simulink model "ARAI_Academy"  (R2020a)
settings: Solver=FixedStepDiscrete  StartTime=0.0  StopTime=10.0  FixedStep=0.02  RelTol=1e-3
InitFcn:
  | mbd_s32k_consistency_checks(bdroot(gcs));
undefined symbols (not defined in the file): Cells_in_Series, LQFP, Temp_in_Series, ts
libraries: hdlsllib x280, mbd_s32k1xx_ec_toolbox x39, simulink x3
(part 1 of 3)
settings Model: Creator=tg-gr  LastModifiedBy=tg-gr
settings DataIOCC: ExternalInput=off  InitialState=off  SaveOutput=off  SignalLogging=off  SaveTime=off
settings OptimizationCC: DefaultParameterBehavior=Inlined  EnhancedBackFolding=on  PassReuseOutputArgsAs=Individual arguments  ZeroExternalMemoryAtStartup=off  ZeroInternalMemoryAtStartup=off  OptimizeBlockOrder=speed  DifferentSizesBufferReuse=on  OptimizationCustomize=off  EfficientTunableParamExpr=on
settings DebuggingCC: InheritedTsInSrcMsg=none  SingleTaskRateTransMsg=error  ParameterTunabilityLossMsg=error  UnconnectedInputMsg=error  UnconnectedOutputMsg=error  UnconnectedLineMsg=error  UnknownTsInhSupMsg=error
settings HardwareCC: ProdBitPerPointer=32  ProdBitPerSizeT=32  ProdBitPerPtrDiffT=32  ProdLargestAtomicInteger=Long  ProdLargestAtomicFloat=Double  ProdWordSize=32  ProdHWDeviceType=ARM Compatible->ARM Cortex
settings SFSimCC: MATLABDynamicMemAlloc=off
settings RTWCC: Description=Model Based Design Toolbox S32K1xx Code Generation Target  SystemTargetFile=mbd_s32k.tlc  MakeCommand=mbd_s32k_make_rtw COPY_MDLREF_INCLUDES=0  TemplateMakefile=mbd_s32k.tmf
settings CodeAppCC: ForceParamTrailComments=on  IgnoreCustomStorageClasses=off  OperatorAnnotations=on  SimulinkDataObjDesc=on  SFDataObjDesc=on  InsertBlockDesc=on
settings STFCustomTargetCC: TargetLangStandard=C99 (ISO)  MultiwordLength=256  CombineOutputUpdateFcns=on  ERTCustomFileBanners=on  SupportContinuousTime=off  SupportNonInlinedSFcns=off  RemoveResetFunc=on  MATLABClassNameForMDSCustomization=Simulink.SoftwareTarget.ERTCustomization  SystemTargetFile=mbd_s32k.tlc
settings ERTTargetCC: TargetLangStandard=C99 (ISO)  ParMdlRefBuildCompliant=off  CompOptLevelCompliant=off  ConcurrentExecutionCompliant=off  ModelStepFunctionPrototypeControlCompliant=off  CPPClassGenCompliant=off  UseToolchainInfoCompliant=off  InlinedParameterPlacement=NonHierarchical  ERTSrcFileBannerTemplate=mbd_ert_code_template.cgt  ERTHdrFileBannerTemplate=mbd_ert_code_template.cgt  ERTDataSrcFileTemplate=mbd_ert_code_template.cgt  ERTDataHdrFileTemplate=mbd_ert_code_template.cgt  ERTCustomFileTemplate=example_file_process.tlc

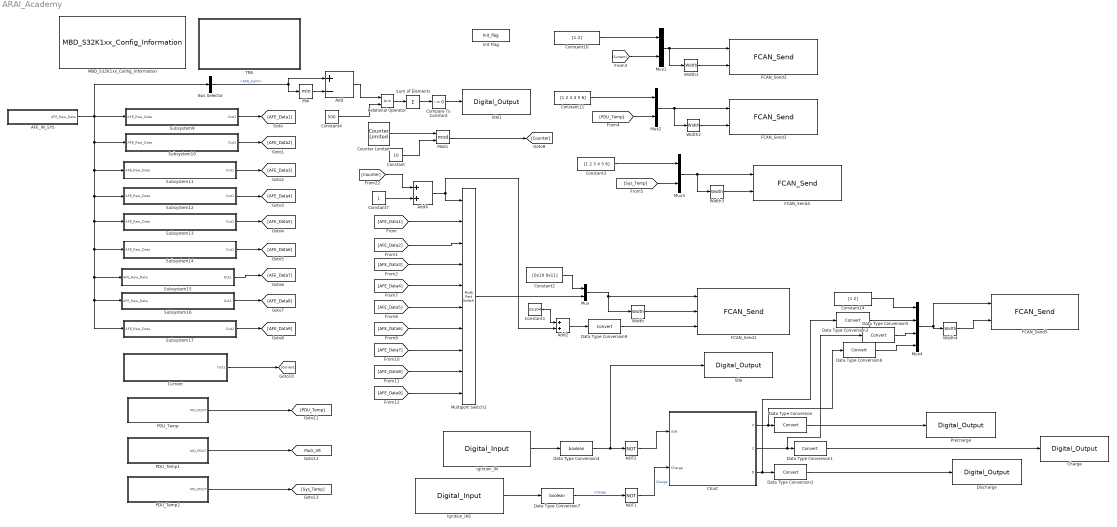
== system ARAI_Academy ==
  AFE_IN_SYS : Subsystem
  Add : Sum  Inputs=+-  OutDataTypeStr=uint16
  Add2 : Sum
  Add4 : Sum
  Bus Selector : BusSelector  OutputSignals=AFE_CellV
  Charge : mbd_s32k1xx_ec_toolbox/GPIO Blocks/Digital_Output  gpio_pin=PTA13: [PTA13 | Port A I/O]  init_val=Low  drive_strength=High
  Chart : Stateflow chart  TreatAsAtomicUnit=on
  Compare To Constant : simulink/Logic and Bit Operations/Compare To Constant  relop=~=  const=0  OutDataTypeStr=boolean
  Constant : Constant  Value=10  OutDataTypeStr=uint8
  Constant1 : Constant  Value=0x104
  Constant10 : Constant  Value=[1 2]  OutDataTypeStr=uint8
  Constant11 : Constant  Value=[1 2 3 4 5 6]  OutDataTypeStr=uint8
  Constant14 : Constant  Value=[1 2]  OutDataTypeStr=uint8
  Constant2 : Constant  Value=[0x10 0x11]
  Constant3 : Constant  Value=[1 2 3 4 5 6]  OutDataTypeStr=uint8
  Constant4 : Constant  Value=500  OutDataTypeStr=uint16
  Constant7 : Constant  OutDataTypeStr=uint8
  Counter Limited : simulink/Sources/Counter Limited  uplimit=8  tsamp=-1
  "Current " : Subsystem
  Data Type Conversion{,1..3,5..6,9} (7 alike) : DataTypeConversion
  Data Type Conversion4 : DataTypeConversion  OutDataTypeStr=boolean
  Data Type Conversion7 : DataTypeConversion  OutDataTypeStr=boolean
  Discharge : mbd_s32k1xx_ec_toolbox/GPIO Blocks/Digital_Output  gpio_pin=PTA12: [PTA12 | Port A I/O]  init_val=Low  drive_strength=High
  FCAN_Send1 : mbd_s32k1xx_ec_toolbox/Communication Blocks/CAN Blocks/FCAN_Send  can_instance=0  can_mode=Non-blocking  can_timeout_ms=0  can_mb_idx=2  can_extended_id=off  can_is_remote=off  can_id=183  show_id_input=on  show_adv_opts=off  can_fd_enable=off  can_enable_brs=off  can_fd_padding=0
  FCAN_Send2 : mbd_s32k1xx_ec_toolbox/Communication Blocks/CAN Blocks/FCAN_Send  can_instance=0  can_mode=Non-blocking  can_timeout_ms=0  can_mb_idx=0  can_extended_id=off  can_is_remote=off  can_id=4  show_id_input=off  show_adv_opts=off  can_fd_enable=off  can_enable_brs=off  can_fd_padding=0
  FCAN_Send3 : mbd_s32k1xx_ec_toolbox/Communication Blocks/CAN Blocks/FCAN_Send  can_instance=0  can_mode=Non-blocking  can_timeout_ms=0  can_mb_idx=1  can_extended_id=off  can_is_remote=off  can_id=1  show_id_input=off  show_adv_opts=off  can_fd_enable=off  can_enable_brs=off  can_fd_padding=0
  FCAN_Send4 : mbd_s32k1xx_ec_toolbox/Communication Blocks/CAN Blocks/FCAN_Send  can_instance=0  can_mode=Non-blocking  can_timeout_ms=0  can_mb_idx=5  can_extended_id=off  can_is_remote=off  can_id=2  show_id_input=off  show_adv_opts=off  can_fd_enable=off  can_enable_brs=off  can_fd_padding=0
  FCAN_Send5 : mbd_s32k1xx_ec_toolbox/Communication Blocks/CAN Blocks/FCAN_Send  can_instance=0  can_mode=Non-blocking  can_timeout_ms=0  can_mb_idx=4  can_extended_id=off  can_is_remote=off  can_id=7  show_id_input=off  show_adv_opts=off  can_fd_enable=off  can_enable_brs=off  can_fd_padding=0
  Idle : mbd_s32k1xx_ec_toolbox/GPIO Blocks/Digital_Output  gpio_pin=PTA11: [PTA11 | Port A I/O]  init_val=Low  drive_strength=High
  Idle1 : mbd_s32k1xx_ec_toolbox/GPIO Blocks/Digital_Output  gpio_pin=PTB9: [PTB9 | Port B I/O]  init_val=Low  drive_strength=High
  Ignition_IN : mbd_s32k1xx_ec_toolbox/GPIO Blocks/Digital_Input  gpio_pin=PTD13: [PTD13 | Port D I/O]  pull_resistor=None  passive_filter=on
  Ignition_IN1 : mbd_s32k1xx_ec_toolbox/GPIO Blocks/Digital_Input  gpio_pin=PTE9: [PTE9 | Port E I/O]  pull_resistor=None  passive_filter=on
  Init Flag : DataStoreMemory  DataStoreName=Init_flag  ReadBeforeWriteMsg=warning  WriteAfterWriteMsg=warning  WriteAfterReadMsg=warning  ShowAdditionalParam=off  OutDataTypeStr=uint8
  MBD_S32K1xx_Config_Information : mbd_s32k1xx_ec_toolbox/MBD_S32K1xx_Config_Information  mbdt_ver=0  disp_str=|  config_params=[]  mcu_target_name=S32K144  mcu_target_package=100-LQFP  mcu_target_sram_size=64KB  mcu_system_clock_freq=80  mcu_xtal_freq=External 8  mcu_steptick_timer=LPIT Channel 0  mcu_steptick_prio=15  ds_import_enable=on  target_compiler=GCC  target_memory=FLASH  gcc_target_compile_opts=-mthumb -mfloat-abi=hard -mfpu=fpv4-sp-d16 -O1 -g -gstrict-dwarf  gcc_target_assemble_opts=-mthumb -mfloat-abi=hard -mfpu=fpv4-sp-d16 -g  gcc_target_link_opts=-mthumb -mfloat-abi=hard -mfpu=fpv4-sp-d16  gcc_target_default_lcf=on  gcc_target_user_lcf=S32K144_64_flash.ld  ghs_target_compile_opts=-cpu=cortexm4f -thumb -fpu=vfpv4_d16 -fsingle -Ogeneral -Wundef -Wimplicit-int -Wshadow -Wtrigraphs --no_commons --gnu_asm -gnu99 -gdwarf-2 -G  ghs_target_assemble_opts=-cpu=cortexm4f -fpu=vfpv4_d16  ghs_target_link_opts=-cpu=cortexm4f -thumb -fpu=vfpv4_d16  ghs_target_default_lcf=on  ghs_target_user_lcf=S32K144_64_flash.ld  iar_target_compile_opts=--cpu=Cortex-M4F --thumb --fpu=VFPv4_sp -Ol -e --debug --dlib_config normal  iar_target_assemble_opts=--cpu Cortex-M4F --thumb --fpu VFPv4_sp  iar_target_link_opts=--no_exceptions --vfe --inline  iar_target_default_lcf=on  iar_target_user_lcf=S32K144_64_flash.icf  pil_download_enable=off  rbl_download_enable=on  rbl_start_delay=5000  rbl_download_interface=OpenSDA  rbl_restart_request=off  rbl_com_port=Custom  rbl_com_port_custom=COM1  pil_download_rate=57600  pil_download_rate_custom=115200  pil_opensda_drive=Custom  pil_opensda_drive_custom=D  jtag_interface=OpenSDA Embedded Debug  pil_uart_instance=1  pil_uart_rx=PTC6: [LPUART1_RX | Receive]  pil_uart_tx=PTC7: [LPUART1_TX | Transmit]  FTM_PWM_PcrCheckEnDis=on  FTM_Input_Edge_Inputs_PcrCheckEnDis=on  FTM_Dual_Edge_Inputs_PcrCheckEnDis=on  FTM_Quadrature_Inputs_PcrCheckEnDis=on  FTM_Hall_Sensor_Inputs_PcrCheckEnDis=on  LPTMR_PcrCheckEnDis=on  PIT_PcrCheckEnDis=on  RTC_PcrCheckEnDis=on  FlexCAN_PcrCheckEnDis=on  LIN_PcrCheckEnDis=on  FlexIO_PcrCheckEnDis=on  LPI2C_PcrCheckEnDis=on  LPSPI_PcrCheckEnDis=on  LPUART_PcrCheckEnDis=on  CMP_PcrCheckEnDis=on  GPIO_OutputPcrCheckEnDis=on  GPIO_InputPcrCheckEnDis=on  SBC_PcrCheckEnDis=on  BMS_PcrCheckEnDis=on  AMMCLIB_PcrCheckEnDis=on  FM_PcrCheckEnDis=on  Profile_PcrCheckEnDis=on  ConfigParams_PcrCheckEnDis=on  ModelRef_PcrCheckEnDis=on  PDB0_PcrCheckEnDis=on  CSEc_PcrCheckEnDis=on  eDMA_PcrCheckEnDis=on  FLASH_PcrCheckEnDis=on  ADC_PcrCheckEnDis=on  WDOG_PcrCheckEnDis=on
      | Target : S32K144-64KB_SRAM
      | Package : 100-pin
      | System clock : 80 MHz
      | XTAL clock : External 8 MHz
      | Compiler : IAR
      | Target Type : FLASH
      | Download Code after build : off
      | Step Tick Interrupt Priority : 15
  Min : MinMax
  Mod1 : Math  Operator=mod  SaturateOnIntegerOverflow=on
  Multiport Switch2 : MultiPortSwitch  Inputs=9  DiagnosticForDefault=None
  Mux{,1..3} (4 alike) : Mux  Inputs=2
  Mux4 : Mux
  NOT1 : Logic  Operator=NOT  IconShape=distinctive  AllPortsSameDT=off  OutDataTypeStr=boolean
  NOT2 : Logic  Operator=NOT  IconShape=distinctive  AllPortsSameDT=off  OutDataTypeStr=boolean
  PDU_Temp : Subsystem
  PDU_Temp1 : Subsystem
  PDU_Temp2 : Subsystem
  Precharge : mbd_s32k1xx_ec_toolbox/GPIO Blocks/Digital_Output  gpio_pin=PTA14: [PTA14 | Port A I/O]  init_val=Low  drive_strength=High
  Relational Operator : RelationalOperator  OutDataTypeStr=boolean  RndMeth=Simplest
  Subsystem10 : Subsystem
  Subsystem11 : Subsystem
  Subsystem12 : Subsystem
  Subsystem13 : Subsystem
  Subsystem14 : Subsystem
  Subsystem15 : Subsystem
  Subsystem16 : Subsystem
  Subsystem17 : Subsystem
  Subsystem9 : Subsystem
  Sum of Elements : Sum  Inputs=+
  TNS : Subsystem  Priority=0
  Width{,1..4} (5 alike) : Width  DataType=uint8
  tag scope: Pack_Vlt=global
  wires:
  Subsystem11/1(Out1) -> [AFE_Data3]
  Subsystem17/1(Out2) -> [AFE_Data9]
  Subsystem16/1(Out1) -> [AFE_Data8]
  Subsystem12/1(Out1) -> [AFE_Data4]
  Subsystem15/1(Out1) -> [AFE_Data7]
  Subsystem13/1(Out1) -> [AFE_Data5]
  Subsystem10/1(Out1) -> [AFE_Data2]
  Subsystem14/1(Out1) -> [AFE_Data6]
  Subsystem9/1(Out1) -> [AFE_Data1]
  AFE_IN_SYS/1(AFE_Raw_Data) -> Subsystem17/1(AFE_Raw_Data), Subsystem16/1(AFE_Raw_Data), Subsystem15/1(AFE_Raw_Data), Subsystem14/1(AFE_Raw_Data), Subsystem13/1(AFE_Raw_Data), Subsystem12/1(AFE_Raw_Data), Subsystem11/1(AFE_Raw_Data), Subsystem10/1(AFE_Raw_Data), Bus Selector/1, Subsystem9/1(AFE_Raw_Data)
  Constant7/1 -> Add4/2
  Add4/1 -> Add2/2, Multiport Switch2/1
  [Counter] -> Add4/1
  [AFE_Data7] -> Multiport Switch2/8
  [AFE_Data9] -> Multiport Switch2/10
  [AFE_Data3] -> Multiport Switch2/4
  Multiport Switch2/1 -> Mux/2
  [AFE_Data5] -> Multiport Switch2/6
  [AFE_Data2] -> Multiport Switch2/3
  Constant2/1 -> Mux/1
  [AFE_Data4] -> Multiport Switch2/5
  [AFE_Data8] -> Multiport Switch2/9
  Data Type Conversion9/1 -> FCAN_Send1/3
  Width/1 -> FCAN_Send1/2
  Mux/1 -> Width/1, FCAN_Send1/1
  [AFE_Data6] -> Multiport Switch2/7
  Add2/1 -> Data Type Conversion9/1
  [AFE_Data1] -> Multiport Switch2/2
  Constant1/1 -> Add2/1
  Constant/1 -> Mod1/2
  Mod1/1 -> [Counter]
  Counter Limited/1 -> Mod1/1
  Mux1/1 -> Width1/1, FCAN_Send2/1
  Width1/1 -> FCAN_Send2/2
  Constant10/1 -> Mux1/1
  Constant11/1 -> Mux2/1
  Width2/1 -> FCAN_Send3/2
  Mux2/1 -> Width2/1, FCAN_Send3/1
  Constant14/1 -> Mux4/1
  Mux4/1 -> FCAN_Send5/1, Width4/1
  Width4/1 -> FCAN_Send5/2
  [Current] -> Mux1/2
  "Current "/1(Out1) -> [Current]
  [PDU_Temp] -> Mux2/2
  PDU_Temp/1(MO_PDUT) -> [PDU_Temp]
  Ignition_IN/1 -> Data Type Conversion4/1
  Chart/1(P) -> Data Type Conversion6/1, Data Type Conversion/1
  Chart/3(D) -> Data Type Conversion3/1, Data Type Conversion2/1
  Chart/2(C) -> Data Type Conversion5/1, Data Type Conversion1/1
  Data Type Conversion/1 -> Precharge/1
  Data Type Conversion3/1 -> Mux4/2
  Data Type Conversion5/1 -> Mux4/3
  Data Type Conversion6/1 -> Mux4/4
  Data Type Conversion1/1 -> Charge/1
  Ignition_IN1/1 -> Data Type Conversion7/1
  NOT1/1 -> Chart/2(Charge)  "Charge"
  Data Type Conversion4/1 -> NOT2/1, Idle/1
  PDU_Temp1/1(MO_PDUT) -> [Pack_Vlt]
  PDU_Temp2/1(MO_PDUT) -> [Sys_Temp]
  [Sys_Temp] -> Mux3/2
  Mux3/1 -> FCAN_Send4/1, Width3/1
  Width3/1 -> FCAN_Send4/2
  Constant3/1 -> Mux3/1
  Add/1 -> Relational Operator/1
  Relational Operator/1 -> Sum of Elements/1
  Constant4/1 -> Relational Operator/2
  Bus Selector/1 -> Add/1, Min/1  "<AFE_CellV>"
  Min/1 -> Add/2
  Sum of Elements/1 -> Compare To Constant/1
  Compare To Constant/1 -> Idle1/1
  Data Type Conversion2/1 -> Discharge/1
  NOT2/1 -> Chart/1(IGN)
  Data Type Conversion7/1 -> NOT1/1  "Charge"

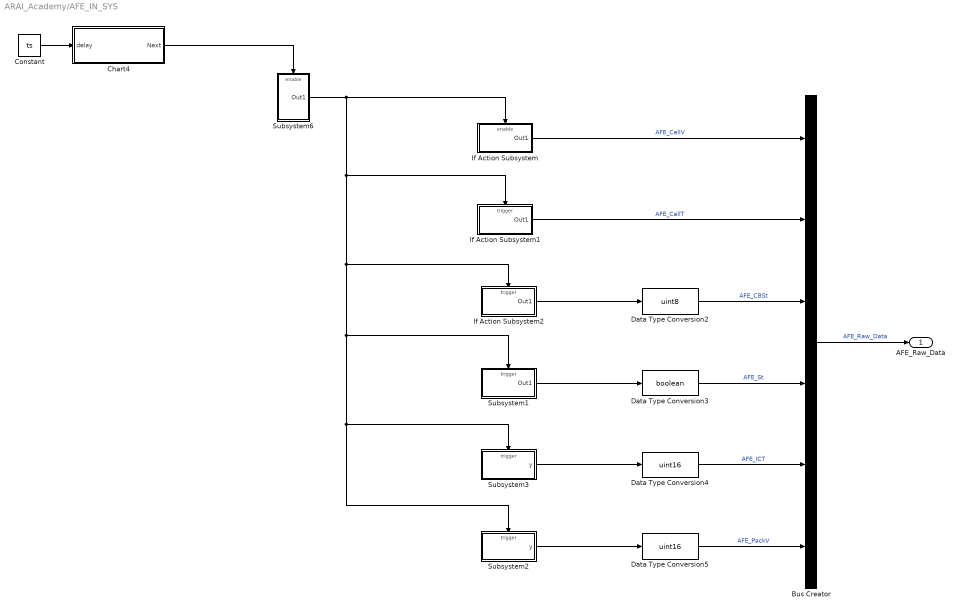
== system ARAI_Academy/AFE_IN_SYS ==
  Bus Creator : BusCreator  Inputs=6
  Chart4 : Stateflow chart  TreatAsAtomicUnit=on
  Constant : Constant  Value=ts
  Data Type Conversion2 : DataTypeConversion  OutDataTypeStr=uint8
  Data Type Conversion3 : DataTypeConversion  OutDataTypeStr=boolean
  Data Type Conversion4 : DataTypeConversion  OutDataTypeStr=uint16
  Data Type Conversion5 : DataTypeConversion  OutDataTypeStr=uint16
  If Action Subsystem : Subsystem  TreatAsAtomicUnit=on
  If Action Subsystem1 : Subsystem  TreatAsAtomicUnit=on
  If Action Subsystem2 : Subsystem  TreatAsAtomicUnit=on
  Subsystem1 : Subsystem
  Subsystem2 : Subsystem
  Subsystem3 : Subsystem
  Subsystem6 : Subsystem
  AFE_Raw_Data : Outport
  wires:
  Subsystem2/1(y) -> Data Type Conversion5/1
  Subsystem3/1(y) -> Data Type Conversion4/1
  Subsystem1/1(Out1) -> Data Type Conversion3/1
  If Action Subsystem2/1(Out1) -> Data Type Conversion2/1
  Data Type Conversion5/1 -> Bus Creator/6  "AFE_PackV"
  Data Type Conversion2/1 -> Bus Creator/3  "AFE_CBSt"
  Data Type Conversion3/1 -> Bus Creator/4  "AFE_St"
  Data Type Conversion4/1 -> Bus Creator/5  "AFE_ICT"
  If Action Subsystem/1(Out1) -> Bus Creator/1  "AFE_CellV"
  If Action Subsystem1/1(Out1) -> Bus Creator/2  "AFE_CellT"
  Bus Creator/1 -> AFE_Raw_Data/1  "AFE_Raw_Data"
  Constant/1 -> Chart4/1(delay)
  Chart4/1(Next) -> Subsystem6/Enable
  Subsystem6/1(Out1) -> If Action Subsystem/Enable, If Action Subsystem1/Trigger, If Action Subsystem2/Trigger, Subsystem1/Trigger, Subsystem3/Trigger, Subsystem2/Trigger

== system ARAI_Academy/Current  ==
  1-D Lookup Table : Lookup_n-D  NumberOfTableDimensions=1  BreakpointsForDimension1=[0 4096]  Table=[-100 100]  ExtrapMethod=Clip  InternalRulePriority=Speed  OutDataTypeStr=int16  RndMeth=Simplest  InputSameDT=on
  CURR_SHT : mbd_s32k1xx_ec_toolbox/Motor Control Blocks/ADC Blocks/ADC_Start  instance=1  adc_r=A  adc_chan=PTB13: [ADC1_SE8 | ADC Single Ended Input]  aien=off  mcuTargetUpdate=on
  Data Type Conversion : DataTypeConversion
  Data Type Conversion3 : DataTypeConversion  OutDataTypeStr=uint16
  Demux : Demux  Outputs=[1 3]
  Saturation : Saturate  UpperLimit=100  LowerLimit=-100
  Subsystem8 : Subsystem
  Terminator1 : Terminator
  Out1 : Outport
  wires:
  CURR_SHT/1 -> Data Type Conversion3/1
  Data Type Conversion3/1 -> 1-D Lookup Table/1
  Demux/2 -> Out1/1
  Demux/1 -> Terminator1/1
  1-D Lookup Table/1 -> Saturation/1
  Subsystem8/1(MO_Current) -> Demux/1  "Val_PackV"
  Data Type Conversion/1 -> Subsystem8/1(In1)
  Saturation/1 -> Data Type Conversion/1

== system ARAI_Academy/PDU_Temp ==
  1-D Lookup Table : Lookup_n-D  NumberOfTableDimensions=1  BreakpointsForDimension1=[0 4096]  Table=[0 70]  ExtrapMethod=Clip  InternalRulePriority=Speed  RndMeth=Simplest  InputSameDT=on
  Data Type Conversion1 : DataTypeConversion  OutDataTypeStr=uint16
  Gain : Gain  Gain=10
  PDU_TP : mbd_s32k1xx_ec_toolbox/Motor Control Blocks/ADC Blocks/ADC_Start  instance=1  adc_r=A  adc_chan=PTD4: [ADC1_SE6 | ADC Single Ended Input]  aien=off  mcuTargetUpdate=on
  Subsystem1 : Subsystem
  MO_PDUT : Outport
  wires:
  1-D Lookup Table/1 -> Gain/1
  PDU_TP/1 -> Data Type Conversion1/1
  Subsystem1/1(MO_PDUT) -> MO_PDUT/1
  Data Type Conversion1/1 -> 1-D Lookup Table/1
  Gain/1 -> Subsystem1/1(In1)

== system ARAI_Academy/PDU_Temp1 ==
  1-D Lookup Table : Lookup_n-D  NumberOfTableDimensions=1  BreakpointsForDimension1=[0 4096]  Table=[39 58]  ExtrapMethod=Clip  InternalRulePriority=Speed  RndMeth=Simplest  InputSameDT=on
  Data Type Conversion1 : DataTypeConversion  OutDataTypeStr=uint16
  Gain : Gain  Gain=100
  PDU_TP : mbd_s32k1xx_ec_toolbox/Motor Control Blocks/ADC Blocks/ADC_Start  instance=0  adc_r=A  adc_chan=PTB3: [ADC0_SE7 | ADC Single Ended Input]  aien=off  mcuTargetUpdate=on
  MO_PDUT : Outport
  wires:
  Data Type Conversion1/1 -> 1-D Lookup Table/1
  1-D Lookup Table/1 -> Gain/1
  PDU_TP/1 -> Data Type Conversion1/1
  Gain/1 -> MO_PDUT/1

== system ARAI_Academy/PDU_Temp2 ==
  1-D Lookup Table : Lookup_n-D  NumberOfTableDimensions=1  BreakpointsForDimension1=[0 4096]  Table=[0 70]  ExtrapMethod=Clip  InternalRulePriority=Speed  RndMeth=Simplest  InputSameDT=on
  Data Type Conversion1 : DataTypeConversion  OutDataTypeStr=uint16
  Gain : Gain  Gain=10
  PDU_TP : mbd_s32k1xx_ec_toolbox/Motor Control Blocks/ADC Blocks/ADC_Start  instance=0  adc_r=A  adc_chan=PTB2: [ADC0_SE6 | ADC Single Ended Input]  aien=off  mcuTargetUpdate=on
  Subsystem1 : Subsystem
  MO_PDUT : Outport
  wires:
  1-D Lookup Table/1 -> Gain/1
  PDU_TP/1 -> Data Type Conversion1/1
  Subsystem1/1(MO_PDUT) -> MO_PDUT/1
  Data Type Conversion1/1 -> 1-D Lookup Table/1
  Gain/1 -> Subsystem1/1(In1)

== system ARAI_Academy/Subsystem10 ==
  AFE_Raw_Data : Inport
  Bus Selector : BusSelector  OutputSignals=AFE_CellV
  Selector : Selector  InputPortWidth=Cells_in_Series*2  IndexOptions=Starting index (dialog)  Indices=7  OutputSizes=6
  Subsystem : Subsystem
  Out1 : Outport
  wires:
  Bus Selector/1 -> Subsystem/1(In1)  "<AFE_CellV>"
  AFE_Raw_Data/1 -> Bus Selector/1
  Selector/1 -> Out1/1
  Subsystem/1(MO_CV_FLT) -> Selector/1

== system ARAI_Academy/Subsystem11 ==
  AFE_Raw_Data : Inport
  Bus Selector : BusSelector  OutputSignals=AFE_CellV
  Selector : Selector  InputPortWidth=Cells_in_Series*2  IndexOptions=Starting index (dialog)  Indices=13  OutputSizes=6
  Subsystem : Subsystem
  Out1 : Outport
  wires:
  Selector/1 -> Out1/1
  AFE_Raw_Data/1 -> Bus Selector/1
  Bus Selector/1 -> Subsystem/1(In1)  "<AFE_CellV>"
  Subsystem/1(MO_CV_FLT) -> Selector/1

== system ARAI_Academy/Subsystem12 ==
  AFE_Raw_Data : Inport
  Bus Selector : BusSelector  OutputSignals=AFE_CellV
  Selector : Selector  InputPortWidth=Cells_in_Series*2  IndexOptions=Starting index (dialog)  Indices=19  OutputSizes=6
  Subsystem : Subsystem
  Out1 : Outport
  wires:
  Bus Selector/1 -> Subsystem/1(In1)  "<AFE_CellV>"
  AFE_Raw_Data/1 -> Bus Selector/1
  Selector/1 -> Out1/1
  Subsystem/1(MO_CV_FLT) -> Selector/1

== system ARAI_Academy/Subsystem13 ==
  AFE_Raw_Data : Inport
  Bus Selector : BusSelector  OutputSignals=AFE_CellV
  Selector : Selector  InputPortWidth=Cells_in_Series*2  IndexOptions=Starting index (dialog)  Indices=25  OutputSizes=6
  Subsystem : Subsystem
  Out1 : Outport
  wires:
  Selector/1 -> Out1/1
  AFE_Raw_Data/1 -> Bus Selector/1
  Bus Selector/1 -> Subsystem/1(In1)  "<AFE_CellV>"
  Subsystem/1(MO_CV_FLT) -> Selector/1

== system ARAI_Academy/Subsystem14 ==
  AFE_Raw_Data : Inport
  Bus Selector : BusSelector  OutputSignals=AFE_CellV,AFE_CellT
  Mux : Mux  Inputs=2.
  Selector : Selector  InputPortWidth=Cells_in_Series*2  IndexOptions=Starting index (dialog)  Indices=31  OutputSizes=2
  Selector2 : Selector  InputPortWidth=Temp_in_Series*2  IndexOptions=Starting index (dialog)  Indices=1  OutputSizes=4
  Subsystem : Subsystem
  Subsystem8 : Subsystem
  Out1 : Outport
  wires:
  Selector2/1 -> Mux/2
  AFE_Raw_Data/1 -> Bus Selector/1
  Mux/1 -> Out1/1
  Selector/1 -> Mux/1
  Bus Selector/1 -> Subsystem/1(In1)  "<AFE_CellV>"
  Bus Selector/2 -> Subsystem8/1(In1)  "<AFE_CellT>"
  Subsystem/1(MO_CV_FLT) -> Selector/1
  Subsystem8/1(MO_CT_FLT) -> Selector2/1  "Val_PDUT"

== system ARAI_Academy/Subsystem15 ==
  AFE_Raw_Data : Inport
  Bus Selector : BusSelector  OutputSignals=AFE_CellT
  Selector : Selector  InputPortWidth=Temp_in_Series*2  IndexOptions=Starting index (dialog)  Indices=5  OutputSizes=6
  Subsystem12 : Subsystem
  Out1 : Outport
  wires:
  Bus Selector/1 -> Subsystem12/1(In1)  "<AFE_CellT>"
  AFE_Raw_Data/1 -> Bus Selector/1
  Selector/1 -> Out1/1
  Subsystem12/1(MO_CT_FLT) -> Selector/1  "Val_PDUT"

== system ARAI_Academy/Subsystem16 ==
  AFE_Raw_Data : Inport
  Bus Selector : BusSelector  OutputSignals=AFE_CellT
  Selector : Selector  InputPortWidth=Temp_in_Series*2  IndexOptions=Starting index (dialog)  Indices=11  OutputSizes=6
  Subsystem12 : Subsystem
  Out1 : Outport
  wires:
  Selector/1 -> Out1/1
  AFE_Raw_Data/1 -> Bus Selector/1
  Bus Selector/1 -> Subsystem12/1(In1)  "<AFE_CellT>"
  Subsystem12/1(MO_CT_FLT) -> Selector/1  "Val_PDUT"

== system ARAI_Academy/Subsystem17 ==
  AFE_Raw_Data : Inport
  Bus Selector : BusSelector  OutputSignals=AFE_ICT,AFE_PackV,AFE_CBSt
  Data Type Conversion : DataTypeConversion
  Mux : Mux  Inputs=3
  Subsystem1 : Subsystem
  Subsystem9 : Subsystem
  Terminator : Terminator
  Out2 : Outport
  wires:
  AFE_Raw_Data/1 -> Bus Selector/1
  Mux/1 -> Out2/1
  Bus Selector/1 -> Subsystem9/1(HI_ICT_Raw)  "<AFE_ICT>"
  Bus Selector/3 -> Data Type Conversion/1  "<AFE_CBSt>"
  Data Type Conversion/1 -> Mux/3
  Subsystem9/1(MO_ICT) -> Mux/1  "ICTemp"
  Subsystem1/1(MO_MaxCellV) -> Mux/2
  [Pack_Vlt] -> Subsystem1/1(In1)
  Bus Selector/2 -> Terminator/1  "<AFE_PackV>"

== system ARAI_Academy/Subsystem9 ==
  AFE_Raw_Data : Inport
  Bus Selector : BusSelector  OutputSignals=AFE_CellV
  Selector6 : Selector  InputPortWidth=Cells_in_Series*2  IndexOptions=Starting index (dialog)  Indices=1  OutputSizes=6
  Subsystem : Subsystem
  Out1 : Outport
  wires:
  AFE_Raw_Data/1 -> Bus Selector/1
  Bus Selector/1 -> Subsystem/1(In1)  "<AFE_CellV>"
  Selector6/1 -> Out1/1
  Subsystem/1(MO_CV_FLT) -> Selector6/1

== system ARAI_Academy/TNS ==
  ADC : Subsystem
  Blink : Stateflow chart  TreatAsAtomicUnit=on
  CAN : Subsystem
  CAN_Supply_EN : mbd_s32k1xx_ec_toolbox/GPIO Blocks/Digital_Output  gpio_pin=PTD8: [PTD8 | Port D I/O]  init_val=Low  drive_strength=High
  Constant3 : Constant  OutDataTypeStr=boolean  SampleTime=-1
  I2C : Subsystem
  LED : mbd_s32k1xx_ec_toolbox/GPIO Blocks/Digital_Output  gpio_pin=PTE14: [PTE14 | Port E I/O]  init_val=Low  drive_strength=Low
  System Outputs : Subsystem  mask(System Outputs){ShowInLibBrowser=0}
      mask prompts: ShowInLibBrowser "Simulink:masks:CustCodeMaskParam1_MP"
      settings: CopyFcn=cccopyfcn(gcb)  OpenFcn=ccopenfcn('System Outputs Function')
      mask Help: eval('feval(''rtwprivate'',''rtwhelpview'',''rtw_sys_outputs_block'')');
      mask DialogControl ShowInLibBrowser Prompt: Mask Parameter 1:
      mask Display: disp('System\nOutputs');
  wires:
  Blink/1(" A") -> LED/1
  Constant3/1 -> CAN_Supply_EN/1

== system ARAI_Academy/AFE_IN_SYS/Chart4/CONFIG_UPDATE_0x0090 ==
  f : TriggerPort  TriggerType=function-call  VariantControl=(inherit)
      settings: CopyFcn=Stateflow.SLINSF.SimulinkMan.removeBlockPreDeleteFcn  PreDeleteFcn=Stateflow.SLINSF.SimulinkMan.unsafePredeleteFcn
  Constant : Constant  Value=[0x3E 0x90 0x00]  OutDataTypeStr=uint8
  Constant1 : Constant  Value=true  OutDataTypeStr=boolean
  Constant2 : Constant  Value=8  OutDataTypeStr=uint16
  LPI2C_Master_Transmit : mbd_s32k1xx_ec_toolbox/Communication Blocks/I2C Blocks/LPI2C_Master_Transmit  instance=0  xfermode=Blocking  Timeout=10  is10bit=off
  wires:
  Constant2/1 -> LPI2C_Master_Transmit/3
  Constant1/1 -> LPI2C_Master_Transmit/2
  Constant/1 -> LPI2C_Master_Transmit/1

== system ARAI_Academy/AFE_IN_SYS/Chart4/Checksum_0x91EA ==
  f : TriggerPort  TriggerType=function-call  VariantControl=(inherit)
      settings: CopyFcn=Stateflow.SLINSF.SimulinkMan.removeBlockPreDeleteFcn  PreDeleteFcn=Stateflow.SLINSF.SimulinkMan.unsafePredeleteFcn
  Constant : Constant  Value=[0x60 0x15 0x18]  OutDataTypeStr=uint8
  Constant1 : Constant  Value=true  OutDataTypeStr=boolean
  Constant2 : Constant  Value=8  OutDataTypeStr=uint16
  LPI2C_Master_Transmit : mbd_s32k1xx_ec_toolbox/Communication Blocks/I2C Blocks/LPI2C_Master_Transmit  instance=0  xfermode=Blocking  Timeout=10  is10bit=off
  wires:
  Constant2/1 -> LPI2C_Master_Transmit/3
  Constant1/1 -> LPI2C_Master_Transmit/2
  Constant/1 -> LPI2C_Master_Transmit/1

== system ARAI_Academy/AFE_IN_SYS/Chart4/Checksum_0x92FA ==
  f : TriggerPort  TriggerType=function-call  VariantControl=(inherit)
      settings: CopyFcn=Stateflow.SLINSF.SimulinkMan.removeBlockPreDeleteFcn  PreDeleteFcn=Stateflow.SLINSF.SimulinkMan.unsafePredeleteFcn
  Constant : Constant  Value=[0x60 0x10 0x0D]  OutDataTypeStr=uint8
  Constant1 : Constant  Value=true  OutDataTypeStr=boolean
  Constant2 : Constant  Value=8  OutDataTypeStr=uint16
  LPI2C_Master_Transmit : mbd_s32k1xx_ec_toolbox/Communication Blocks/I2C Blocks/LPI2C_Master_Transmit  instance=0  xfermode=Blocking  Timeout=10  is10bit=off
  wires:
  Constant2/1 -> LPI2C_Master_Transmit/3
  Constant1/1 -> LPI2C_Master_Transmit/2
  Constant/1 -> LPI2C_Master_Transmit/1

== system ARAI_Academy/AFE_IN_SYS/Chart4/Checksum_0x9335 ==
  f : TriggerPort  TriggerType=function-call  VariantControl=(inherit)
      settings: CopyFcn=Stateflow.SLINSF.SimulinkMan.removeBlockPreDeleteFcn  PreDeleteFcn=Stateflow.SLINSF.SimulinkMan.unsafePredeleteFcn
  Constant : Constant  Value=[0x60 0x37 0x05]  OutDataTypeStr=uint8
  Constant1 : Constant  Value=true  OutDataTypeStr=boolean
  Constant2 : Constant  Value=8  OutDataTypeStr=uint16
  LPI2C_Master_Transmit : mbd_s32k1xx_ec_toolbox/Communication Blocks/I2C Blocks/LPI2C_Master_Transmit  instance=0  xfermode=Blocking  Timeout=10  is10bit=off
  wires:
  Constant2/1 -> LPI2C_Master_Transmit/3
  Constant1/1 -> LPI2C_Master_Transmit/2
  Constant/1 -> LPI2C_Master_Transmit/1

== system ARAI_Academy/AFE_IN_SYS/Chart4/Checksum_0x9339 ==
  f : TriggerPort  TriggerType=function-call  VariantControl=(inherit)
      settings: CopyFcn=Stateflow.SLINSF.SimulinkMan.removeBlockPreDeleteFcn  PreDeleteFcn=Stateflow.SLINSF.SimulinkMan.unsafePredeleteFcn
  Constant : Constant  Value=[0x60 0xF7 0x05]  OutDataTypeStr=uint8
  Constant1 : Constant  Value=true  OutDataTypeStr=boolean
  Constant2 : Constant  Value=8  OutDataTypeStr=uint16
  LPI2C_Master_Transmit : mbd_s32k1xx_ec_toolbox/Communication Blocks/I2C Blocks/LPI2C_Master_Transmit  instance=0  xfermode=Blocking  Timeout=10  is10bit=off
  wires:
  Constant2/1 -> LPI2C_Master_Transmit/3
  Constant1/1 -> LPI2C_Master_Transmit/2
  Constant/1 -> LPI2C_Master_Transmit/1

== system ARAI_Academy/AFE_IN_SYS/Chart4/EXIT_CFGUPDATE_0x9200 ==
  f : TriggerPort  TriggerType=function-call  VariantControl=(inherit)
      settings: CopyFcn=Stateflow.SLINSF.SimulinkMan.removeBlockPreDeleteFcn  PreDeleteFcn=Stateflow.SLINSF.SimulinkMan.unsafePredeleteFcn
  Constant : Constant  Value=[0x3E 0x92 0x00]  OutDataTypeStr=uint8
  Constant1 : Constant  Value=true  OutDataTypeStr=boolean
  Constant2 : Constant  Value=8  OutDataTypeStr=uint16
  LPI2C_Master_Transmit : mbd_s32k1xx_ec_toolbox/Communication Blocks/I2C Blocks/LPI2C_Master_Transmit  instance=0  xfermode=Blocking  Timeout=10  is10bit=off
  wires:
  Constant1/1 -> LPI2C_Master_Transmit/2
  Constant/1 -> LPI2C_Master_Transmit/1
  Constant2/1 -> LPI2C_Master_Transmit/3

== system ARAI_Academy/AFE_IN_SYS/Chart4/Pin_Confi_0x91EA ==
  f : TriggerPort  TriggerType=function-call  VariantControl=(inherit)
      settings: CopyFcn=Stateflow.SLINSF.SimulinkMan.removeBlockPreDeleteFcn  PreDeleteFcn=Stateflow.SLINSF.SimulinkMan.unsafePredeleteFcn
  Constant : Constant  Value=[0x3E 0xEA 0x91 0xF4 0xBE 0x52 0x71 0xF8 0xA9 0xD4 0x66 0x3F 0x05 0x45 0xF0 0x4D 0x16 0x72 0xEE 0xEE 0x11 0xB7 0x2D]  OutDataTypeStr=uint8
  Constant1 : Constant  Value=true  OutDataTypeStr=boolean
  Constant2 : Constant  Value=8  OutDataTypeStr=uint16
  LPI2C_Master_Transmit : mbd_s32k1xx_ec_toolbox/Communication Blocks/I2C Blocks/LPI2C_Master_Transmit  instance=0  xfermode=Blocking  Timeout=10  is10bit=off
  wires:
  Constant2/1 -> LPI2C_Master_Transmit/3
  Constant1/1 -> LPI2C_Master_Transmit/2
  Constant/1 -> LPI2C_Master_Transmit/1

== system ARAI_Academy/AFE_IN_SYS/Chart4/Pin_Confi_0x92FA ==
  f : TriggerPort  TriggerType=function-call  VariantControl=(inherit)
      settings: CopyFcn=Stateflow.SLINSF.SimulinkMan.removeBlockPreDeleteFcn  PreDeleteFcn=Stateflow.SLINSF.SimulinkMan.unsafePredeleteFcn
  Constant3 : Constant  Value="[0x3E 0xFA 0x92 0x0B  0x0B  0x0B  0x0B  0x0B  0x0B  0x0B  0x0B  0x0B]"  OutDataTypeStr=uint8
  Constant4 : Constant  Value=true  OutDataTypeStr=boolean
  Constant5 : Constant  Value=8  OutDataTypeStr=uint16
  LPI2C_Master_Transmit1 : mbd_s32k1xx_ec_toolbox/Communication Blocks/I2C Blocks/LPI2C_Master_Transmit  instance=0  xfermode=Blocking  Timeout=10  is10bit=off
  wires:
  Constant5/1 -> LPI2C_Master_Transmit1/3
  Constant4/1 -> LPI2C_Master_Transmit1/2
  Constant3/1 -> LPI2C_Master_Transmit1/1

== system ARAI_Academy/AFE_IN_SYS/Chart4/Pin_Confi_0x9335 ==
  f : TriggerPort  TriggerType=function-call  VariantControl=(inherit)
      settings: CopyFcn=Stateflow.SLINSF.SimulinkMan.removeBlockPreDeleteFcn  PreDeleteFcn=Stateflow.SLINSF.SimulinkMan.unsafePredeleteFcn
  Constant : Constant  Value=[0x3E 0x35 0x93 0x00]  OutDataTypeStr=uint8
  Constant1 : Constant  Value=true  OutDataTypeStr=boolean
  Constant2 : Constant  Value=8  OutDataTypeStr=uint16
  LPI2C_Master_Transmit : mbd_s32k1xx_ec_toolbox/Communication Blocks/I2C Blocks/LPI2C_Master_Transmit  instance=0  xfermode=Blocking  Timeout=10  is10bit=off
  wires:
  Constant2/1 -> LPI2C_Master_Transmit/3
  Constant1/1 -> LPI2C_Master_Transmit/2
  Constant/1 -> LPI2C_Master_Transmit/1

== system ARAI_Academy/AFE_IN_SYS/Chart4/Pin_Confi_0x9339 ==
  f : TriggerPort  TriggerType=function-call  VariantControl=(inherit)
      settings: CopyFcn=Stateflow.SLINSF.SimulinkMan.removeBlockPreDeleteFcn  PreDeleteFcn=Stateflow.SLINSF.SimulinkMan.unsafePredeleteFcn
  Constant : Constant  Value=[0x3E 0x39 0x93 0x3C]  OutDataTypeStr=uint8
  Constant1 : Constant  Value=true  OutDataTypeStr=boolean
  Constant2 : Constant  Value=8  OutDataTypeStr=uint16
  LPI2C_Master_Transmit : mbd_s32k1xx_ec_toolbox/Communication Blocks/I2C Blocks/LPI2C_Master_Transmit  instance=0  xfermode=Blocking  Timeout=10  is10bit=off
  wires:
  Constant2/1 -> LPI2C_Master_Transmit/3
  Constant1/1 -> LPI2C_Master_Transmit/2
  Constant/1 -> LPI2C_Master_Transmit/1

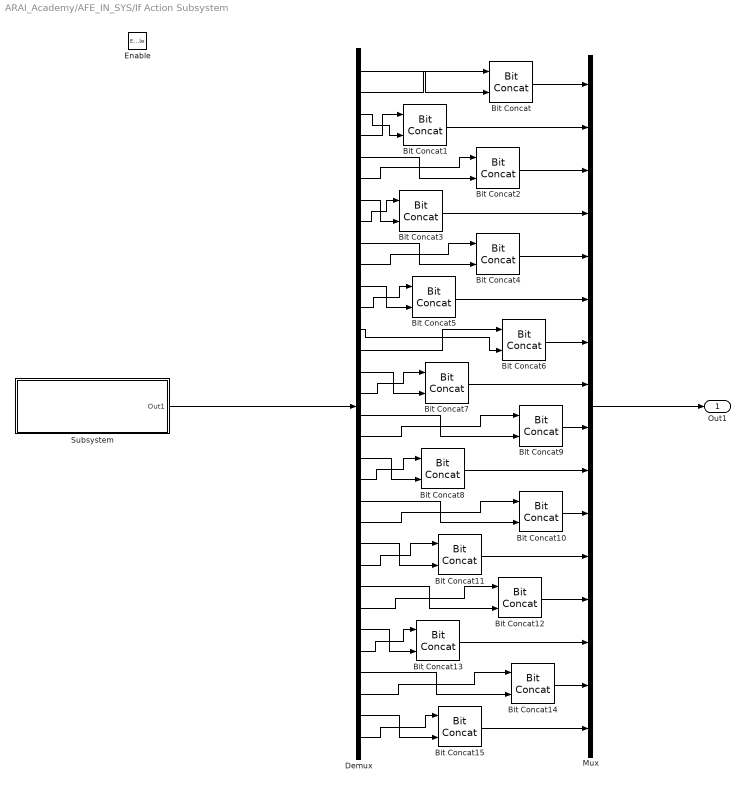
== system ARAI_Academy/AFE_IN_SYS/If Action Subsystem ==
  Enable : EnablePort
  Bit Concat{,1..15} (16 alike) : hdlsllib/Logic and Bit Operations/Bit Concat  numInputs=2
  Demux : Demux  Outputs=32
  Mux : Mux  Inputs=16
  Subsystem : Subsystem
  Out1 : Outport
  wires:
  Bit Concat10/1 -> Mux/11
  Bit Concat15/1 -> Mux/16
  Bit Concat9/1 -> Mux/9
  Bit Concat7/1 -> Mux/8
  Demux/1 -> Bit Concat/2
  Bit Concat5/1 -> Mux/6
  Bit Concat1/1 -> Mux/2
  Bit Concat/1 -> Mux/1
  Bit Concat14/1 -> Mux/15
  Bit Concat12/1 -> Mux/13
  Bit Concat11/1 -> Mux/12
  Demux/4 -> Bit Concat1/1
  Bit Concat6/1 -> Mux/7
  Bit Concat13/1 -> Mux/14
  Bit Concat2/1 -> Mux/3
  Demux/6 -> Bit Concat2/1
  Bit Concat8/1 -> Mux/10
  Demux/3 -> Bit Concat1/2
  Mux/1 -> Out1/1
  Demux/5 -> Bit Concat2/2
  Bit Concat4/1 -> Mux/5
  Bit Concat3/1 -> Mux/4
  Demux/2 -> Bit Concat/1
  Demux/7 -> Bit Concat3/2
  Demux/8 -> Bit Concat3/1
  Demux/9 -> Bit Concat4/2
  Demux/10 -> Bit Concat4/1
  Demux/11 -> Bit Concat5/2
  Demux/12 -> Bit Concat5/1
  Demux/13 -> Bit Concat6/2
  Demux/14 -> Bit Concat6/1
  Demux/15 -> Bit Concat7/2
  Demux/16 -> Bit Concat7/1
  Demux/17 -> Bit Concat9/2
  Demux/18 -> Bit Concat9/1
  Demux/19 -> Bit Concat8/2
  Demux/20 -> Bit Concat8/1
  Demux/21 -> Bit Concat10/2
  Demux/22 -> Bit Concat10/1
  Demux/23 -> Bit Concat11/2
  Demux/24 -> Bit Concat11/1
  Demux/25 -> Bit Concat12/2
  Demux/26 -> Bit Concat12/1
  Demux/27 -> Bit Concat13/2
  Demux/28 -> Bit Concat13/1
  Demux/29 -> Bit Concat14/2
  Demux/30 -> Bit Concat14/1
  Demux/31 -> Bit Concat15/2
  Demux/32 -> Bit Concat15/1
  Subsystem/1(Out1) -> Demux/1

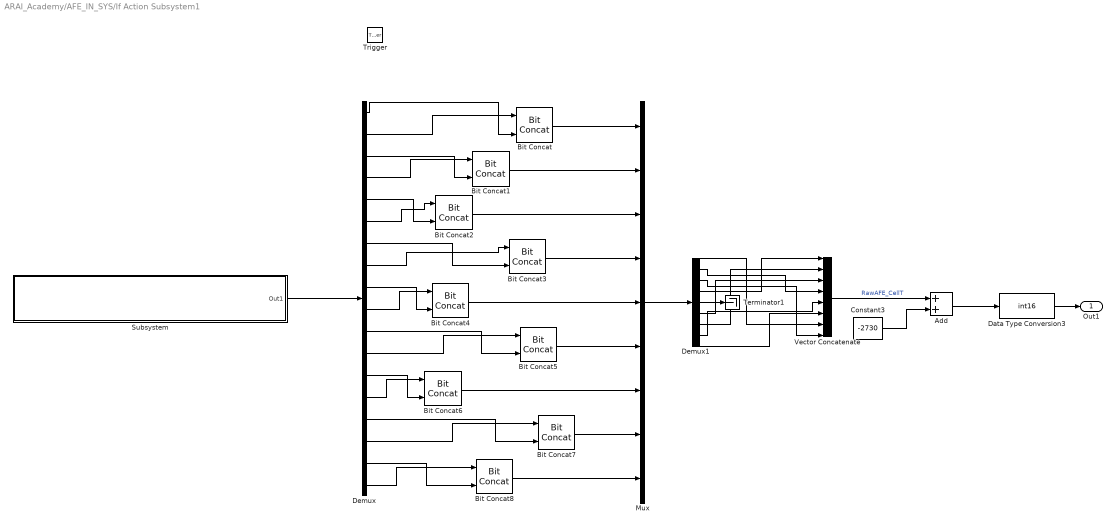
== system ARAI_Academy/AFE_IN_SYS/If Action Subsystem1 ==
  Trigger : TriggerPort  VariantControl=Variant  PortDimensions=1
  Add : Sum
  Bit Concat{,1..8} (9 alike) : hdlsllib/Logic and Bit Operations/Bit Concat  numInputs=2
  Constant3 : Constant  Value=-2730  OutDataTypeStr=int16
  Data Type Conversion3 : DataTypeConversion  OutDataTypeStr=int16
  Demux : Demux  Outputs=18
  Demux1 : Demux  Outputs=9
  Mux : Mux  Inputs=9
  Subsystem : Subsystem
  Terminator1 : Terminator
  Vector Concatenate : Concatenate  NumInputs=8
  Out1 : Outport
  wires:
  Demux/11 -> Bit Concat5/2
  Demux1/9 -> Vector Concatenate/6
  Demux1/7 -> Vector Concatenate/2
  Subsystem/1(Out1) -> Demux/1
  Bit Concat7/1 -> Mux/8
  Mux/1 -> Demux1/1
  Demux1/2 -> Vector Concatenate/4
  Bit Concat4/1 -> Mux/5
  Demux1/8 -> Vector Concatenate/5
  Demux1/3 -> Vector Concatenate/8
  Demux1/5 -> Terminator1/1
  Bit Concat/1 -> Mux/1
  Demux1/6 -> Vector Concatenate/3
  Demux1/1 -> Vector Concatenate/7
  Demux1/4 -> Vector Concatenate/1
  Demux/8 -> Bit Concat3/1
  Demux/7 -> Bit Concat3/2
  Vector Concatenate/1 -> Add/1  "RawAFE_CellT"
  Bit Concat1/1 -> Mux/2
  Demux/14 -> Bit Concat6/1
  Demux/15 -> Bit Concat7/2
  Bit Concat8/1 -> Mux/9
  Bit Concat3/1 -> Mux/4
  Demux/10 -> Bit Concat4/1
  Demux/6 -> Bit Concat2/1
  Demux/2 -> Bit Concat/1
  Demux/1 -> Bit Concat/2
  Demux/5 -> Bit Concat2/2
  Demux/3 -> Bit Concat1/2
  Demux/4 -> Bit Concat1/1
  Demux/16 -> Bit Concat7/1
  Demux/12 -> Bit Concat5/1
  Demux/17 -> Bit Concat8/2
  Demux/18 -> Bit Concat8/1
  Demux/9 -> Bit Concat4/2
  Bit Concat2/1 -> Mux/3
  Bit Concat6/1 -> Mux/7
  Demux/13 -> Bit Concat6/2
  Bit Concat5/1 -> Mux/6
  Constant3/1 -> Add/2
  Add/1 -> Data Type Conversion3/1
  Data Type Conversion3/1 -> Out1/1

== system ARAI_Academy/AFE_IN_SYS/If Action Subsystem2 ==
  Trigger : TriggerPort  VariantControl=Variant  PortDimensions=1
  Constant19 : Constant  Value=0x40  OutDataTypeStr=uint8
  Constant20 : Constant  Value=true  OutDataTypeStr=Inherit: Inherit via back propagation
  Constant21 : Constant  Value=8  OutDataTypeStr=uint16
  Constant22 : Constant  Value=2  OutDataTypeStr=uint32
  LPI2C_Master_Multi_Transfer2 : mbd_s32k1xx_ec_toolbox/Communication Blocks/I2C Blocks/LPI2C_Master_Multi_Transfer  instance=0  xfermode=Blocking  Timeout=3  delay_between_transfers=0  is10bit=off
  Out1 : Outport  PortDimensions=2
  wires:
  LPI2C_Master_Multi_Transfer2/1 -> Out1/1
  Constant21/1 -> LPI2C_Master_Multi_Transfer2/3
  Constant22/1 -> LPI2C_Master_Multi_Transfer2/4
  Constant20/1 -> LPI2C_Master_Multi_Transfer2/2
  Constant19/1 -> LPI2C_Master_Multi_Transfer2/1

== system ARAI_Academy/AFE_IN_SYS/Subsystem1 ==
  Trigger : TriggerPort  VariantControl=Variant  PortDimensions=1
  Constant24 : Constant  Value=0x68  OutDataTypeStr=uint8
  Constant25 : Constant  Value=true  OutDataTypeStr=Inherit: Inherit via back propagation
  Constant26 : Constant  Value=8  OutDataTypeStr=uint16
  Constant27 : Constant  Value=2  OutDataTypeStr=uint32
  LPI2C_Master_Multi_Transfer3 : mbd_s32k1xx_ec_toolbox/Communication Blocks/I2C Blocks/LPI2C_Master_Multi_Transfer  instance=0  xfermode=Blocking  Timeout=3  delay_between_transfers=0  is10bit=off
  Subsystem : Subsystem
  Out1 : Outport
  wires:
  Constant25/1 -> LPI2C_Master_Multi_Transfer3/2
  Constant24/1 -> LPI2C_Master_Multi_Transfer3/1
  Constant27/1 -> LPI2C_Master_Multi_Transfer3/4
  Constant26/1 -> LPI2C_Master_Multi_Transfer3/3
  LPI2C_Master_Multi_Transfer3/1 -> Subsystem/1(In1)
  Subsystem/1(y) -> Out1/1

== system ARAI_Academy/AFE_IN_SYS/Subsystem2 ==
  Trigger : TriggerPort  VariantControl=Variant  PortDimensions=1
  Constant28 : Constant  Value=0x34  OutDataTypeStr=uint8
  Constant29 : Constant  Value=true  OutDataTypeStr=Inherit: Inherit via back propagation
  Constant30 : Constant  Value=8  OutDataTypeStr=uint16
  Constant31 : Constant  Value=2  OutDataTypeStr=uint32
  LPI2C_Master_Multi_Transfer4 : mbd_s32k1xx_ec_toolbox/Communication Blocks/I2C Blocks/LPI2C_Master_Multi_Transfer  instance=0  xfermode=Blocking  Timeout=3  delay_between_transfers=0  is10bit=off
  Subsystem : Subsystem
  y : Outport
  wires:
  Constant30/1 -> LPI2C_Master_Multi_Transfer4/3
  Constant31/1 -> LPI2C_Master_Multi_Transfer4/4
  Constant29/1 -> LPI2C_Master_Multi_Transfer4/2
  Constant28/1 -> LPI2C_Master_Multi_Transfer4/1
  LPI2C_Master_Multi_Transfer4/1 -> Subsystem/1(In1)
  Subsystem/1(y) -> y/1

== system ARAI_Academy/AFE_IN_SYS/Subsystem3 ==
  Trigger : TriggerPort  VariantControl=Variant  PortDimensions=1
  Constant32 : Constant  Value=0x40  OutDataTypeStr=uint8
  Constant33 : Constant  Value=true  OutDataTypeStr=Inherit: Inherit via back propagation
  Constant34 : Constant  Value=8  OutDataTypeStr=uint16
  Constant35 : Constant  Value=2  OutDataTypeStr=uint32
  LPI2C_Master_Multi_Transfer5 : mbd_s32k1xx_ec_toolbox/Communication Blocks/I2C Blocks/LPI2C_Master_Multi_Transfer  Priority=1  instance=0  xfermode=Blocking  Timeout=3  delay_between_transfers=2  is10bit=off
  Subsystem : Subsystem
  y : Outport
  wires:
  Subsystem/1(y) -> y/1
  Constant33/1 -> LPI2C_Master_Multi_Transfer5/2
  Constant35/1 -> LPI2C_Master_Multi_Transfer5/4
  Constant32/1 -> LPI2C_Master_Multi_Transfer5/1
  Constant34/1 -> LPI2C_Master_Multi_Transfer5/3
  LPI2C_Master_Multi_Transfer5/1 -> Subsystem/1(In1)

== system ARAI_Academy/AFE_IN_SYS/Subsystem6 ==
  Enable : EnablePort
  Constant9 : Constant  Value=6  OutDataTypeStr=uint8
  Counter Free-Running1 : simulink/Sources/Counter Free-Running  NumBits=8  tsamp=-1
  Mod : Math  Operator=mod  SaturateOnIntegerOverflow=on
  Out1 : Outport  InitialOutput=10
  wires:
  Constant9/1 -> Mod/2
  Mod/1 -> Out1/1
  Counter Free-Running1/1 -> Mod/1

== system ARAI_Academy/Current /Subsystem8 ==
  In1 : Inport
  Bit Slice : hdlsllib/Logic and Bit Operations/Bit Slice  lidx=15  ridx=8
      settings: SourceProductBaseCode=SL
  Bit Slice1 : hdlsllib/Logic and Bit Operations/Bit Slice  lidx=7  ridx=0
      settings: SourceProductBaseCode=SL
  Bit Slice2 : hdlsllib/Logic and Bit Operations/Bit Slice  lidx=31  ridx=24
      settings: SourceProductBaseCode=SL
  Bit Slice4 : hdlsllib/Logic and Bit Operations/Bit Slice  lidx=23  ridx=16
      settings: SourceProductBaseCode=SL
  Data Type Conversion : DataTypeConversion  OutDataTypeStr=int32
  Gain : Gain  Gain=100
  Mux : Mux
  MO_Current : Outport
  wires:
  Mux/1 -> MO_Current/1
  Bit Slice1/1 -> Mux/4
  Bit Slice/1 -> Mux/3
  In1/1 -> Gain/1
  Bit Slice4/1 -> Mux/2
  Data Type Conversion/1 -> Bit Slice1/1, Bit Slice2/1, Bit Slice4/1, Bit Slice/1
  Gain/1 -> Data Type Conversion/1
  Bit Slice2/1 -> Mux/1

== system ARAI_Academy/PDU_Temp/Subsystem1 ==
  In1 : Inport
  Bit Slice : hdlsllib/Logic and Bit Operations/Bit Slice  lidx=15  ridx=8
      settings: SourceProductBaseCode=SL
  Bit Slice1 : hdlsllib/Logic and Bit Operations/Bit Slice  lidx=7  ridx=0
      settings: SourceProductBaseCode=SL
  Data Type Conversion : DataTypeConversion  OutDataTypeStr=uint16
  Mux : Mux  Inputs=2
  MO_PDUT : Outport
  wires:
  Bit Slice/1 -> Mux/1
  In1/1 -> Data Type Conversion/1
  Bit Slice1/1 -> Mux/2
  Mux/1 -> MO_PDUT/1
  Data Type Conversion/1 -> Bit Slice/1, Bit Slice1/1

== system ARAI_Academy/PDU_Temp2/Subsystem1 ==
  In1 : Inport
  Bit Slice : hdlsllib/Logic and Bit Operations/Bit Slice  lidx=15  ridx=8
      settings: SourceProductBaseCode=SL
  Bit Slice1 : hdlsllib/Logic and Bit Operations/Bit Slice  lidx=7  ridx=0
      settings: SourceProductBaseCode=SL
  Data Type Conversion : DataTypeConversion  OutDataTypeStr=uint16
  Mux : Mux  Inputs=2
  MO_PDUT : Outport
  wires:
  Bit Slice/1 -> Mux/1
  In1/1 -> Data Type Conversion/1
  Bit Slice1/1 -> Mux/2
  Mux/1 -> MO_PDUT/1
  Data Type Conversion/1 -> Bit Slice/1, Bit Slice1/1

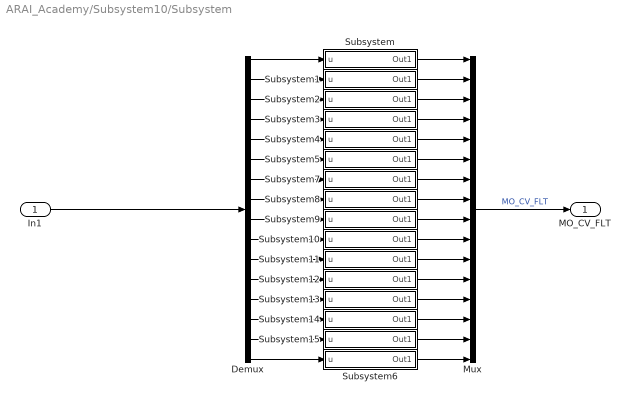
== system ARAI_Academy/Subsystem10/Subsystem ==
  In1 : Inport
  Demux : Demux  Outputs=16
  Mux : Mux  Inputs=16
  Subsystem : Subsystem
  Subsystem1 : Subsystem
  Subsystem10 : Subsystem
  Subsystem11 : Subsystem
  Subsystem12 : Subsystem
  Subsystem13 : Subsystem
  Subsystem14 : Subsystem
  Subsystem15 : Subsystem
  Subsystem2 : Subsystem
  Subsystem3 : Subsystem
  Subsystem4 : Subsystem
  Subsystem5 : Subsystem
  Subsystem6 : Subsystem
  Subsystem7 : Subsystem
  Subsystem8 : Subsystem
  Subsystem9 : Subsystem
  MO_CV_FLT : Outport
  wires:
  In1/1 -> Demux/1
  Demux/1 -> Subsystem/1(u)
  Demux/16 -> Subsystem6/1(u)
  Demux/2 -> Subsystem1/1(u)
  Demux/3 -> Subsystem2/1(u)
  Demux/4 -> Subsystem3/1(u)
  Demux/5 -> Subsystem4/1(u)
  Demux/6 -> Subsystem5/1(u)
  Demux/7 -> Subsystem7/1(u)
  Demux/8 -> Subsystem8/1(u)
  Demux/9 -> Subsystem9/1(u)
  Demux/10 -> Subsystem10/1(u)
  Demux/11 -> Subsystem11/1(u)
  Demux/12 -> Subsystem12/1(u)
  Demux/13 -> Subsystem13/1(u)
  Demux/14 -> Subsystem14/1(u)
  Demux/15 -> Subsystem15/1(u)
  Subsystem/1(Out1) -> Mux/1
  Subsystem1/1(Out1) -> Mux/2
  Subsystem2/1(Out1) -> Mux/3
  Subsystem3/1(Out1) -> Mux/4
  Subsystem4/1(Out1) -> Mux/5
  Subsystem5/1(Out1) -> Mux/6
  Subsystem7/1(Out1) -> Mux/7
  Subsystem8/1(Out1) -> Mux/8
  Subsystem9/1(Out1) -> Mux/9
  Subsystem10/1(Out1) -> Mux/10
  Subsystem11/1(Out1) -> Mux/11
  Subsystem12/1(Out1) -> Mux/12
  Subsystem13/1(Out1) -> Mux/13
  Subsystem14/1(Out1) -> Mux/14
  Subsystem15/1(Out1) -> Mux/15
  Subsystem6/1(Out1) -> Mux/16
  Mux/1 -> MO_CV_FLT/1  "MO_CV_FLT"

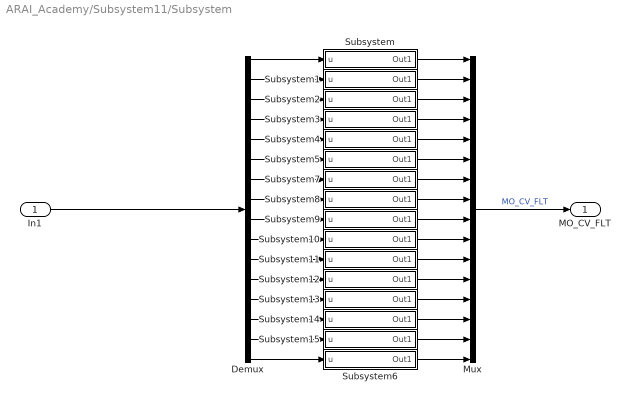
== system ARAI_Academy/Subsystem11/Subsystem ==
  In1 : Inport
  Demux : Demux  Outputs=16
  Mux : Mux  Inputs=16
  Subsystem : Subsystem
  Subsystem1 : Subsystem
  Subsystem10 : Subsystem
  Subsystem11 : Subsystem
  Subsystem12 : Subsystem
  Subsystem13 : Subsystem
  Subsystem14 : Subsystem
  Subsystem15 : Subsystem
  Subsystem2 : Subsystem
  Subsystem3 : Subsystem
  Subsystem4 : Subsystem
  Subsystem5 : Subsystem
  Subsystem6 : Subsystem
  Subsystem7 : Subsystem
  Subsystem8 : Subsystem
  Subsystem9 : Subsystem
  MO_CV_FLT : Outport
  wires:
  In1/1 -> Demux/1
  Demux/1 -> Subsystem/1(u)
  Demux/16 -> Subsystem6/1(u)
  Demux/2 -> Subsystem1/1(u)
  Demux/3 -> Subsystem2/1(u)
  Demux/4 -> Subsystem3/1(u)
  Demux/5 -> Subsystem4/1(u)
  Demux/6 -> Subsystem5/1(u)
  Demux/7 -> Subsystem7/1(u)
  Demux/8 -> Subsystem8/1(u)
  Demux/9 -> Subsystem9/1(u)
  Demux/10 -> Subsystem10/1(u)
  Demux/11 -> Subsystem11/1(u)
  Demux/12 -> Subsystem12/1(u)
  Demux/13 -> Subsystem13/1(u)
  Demux/14 -> Subsystem14/1(u)
  Demux/15 -> Subsystem15/1(u)
  Subsystem/1(Out1) -> Mux/1
  Subsystem1/1(Out1) -> Mux/2
  Subsystem2/1(Out1) -> Mux/3
  Subsystem3/1(Out1) -> Mux/4
  Subsystem4/1(Out1) -> Mux/5
  Subsystem5/1(Out1) -> Mux/6
  Subsystem7/1(Out1) -> Mux/7
  Subsystem8/1(Out1) -> Mux/8
  Subsystem9/1(Out1) -> Mux/9
  Subsystem10/1(Out1) -> Mux/10
  Subsystem11/1(Out1) -> Mux/11
  Subsystem12/1(Out1) -> Mux/12
  Subsystem13/1(Out1) -> Mux/13
  Subsystem14/1(Out1) -> Mux/14
  Subsystem15/1(Out1) -> Mux/15
  Subsystem6/1(Out1) -> Mux/16
  Mux/1 -> MO_CV_FLT/1  "MO_CV_FLT"

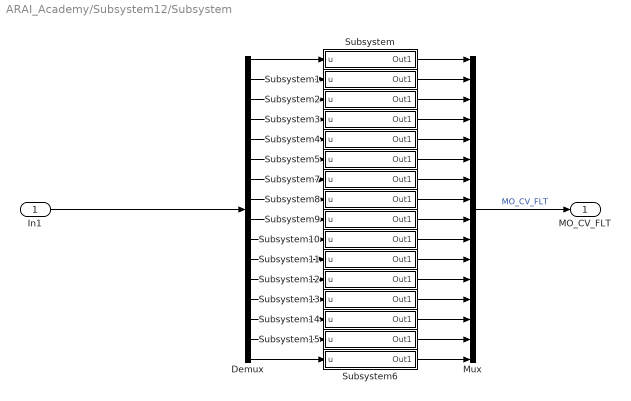
== system ARAI_Academy/Subsystem12/Subsystem ==
  In1 : Inport
  Demux : Demux  Outputs=16
  Mux : Mux  Inputs=16
  Subsystem : Subsystem
  Subsystem1 : Subsystem
  Subsystem10 : Subsystem
  Subsystem11 : Subsystem
  Subsystem12 : Subsystem
  Subsystem13 : Subsystem
  Subsystem14 : Subsystem
  Subsystem15 : Subsystem
  Subsystem2 : Subsystem
  Subsystem3 : Subsystem
  Subsystem4 : Subsystem
  Subsystem5 : Subsystem
  Subsystem6 : Subsystem
  Subsystem7 : Subsystem
  Subsystem8 : Subsystem
  Subsystem9 : Subsystem
  MO_CV_FLT : Outport
  wires:
  In1/1 -> Demux/1
  Demux/1 -> Subsystem/1(u)
  Demux/16 -> Subsystem6/1(u)
  Demux/2 -> Subsystem1/1(u)
  Demux/3 -> Subsystem2/1(u)
  Demux/4 -> Subsystem3/1(u)
  Demux/5 -> Subsystem4/1(u)
  Demux/6 -> Subsystem5/1(u)
  Demux/7 -> Subsystem7/1(u)
  Demux/8 -> Subsystem8/1(u)
  Demux/9 -> Subsystem9/1(u)
  Demux/10 -> Subsystem10/1(u)
  Demux/11 -> Subsystem11/1(u)
  Demux/12 -> Subsystem12/1(u)
  Demux/13 -> Subsystem13/1(u)
  Demux/14 -> Subsystem14/1(u)
  Demux/15 -> Subsystem15/1(u)
  Subsystem/1(Out1) -> Mux/1
  Subsystem1/1(Out1) -> Mux/2
  Subsystem2/1(Out1) -> Mux/3
  Subsystem3/1(Out1) -> Mux/4
  Subsystem4/1(Out1) -> Mux/5
  Subsystem5/1(Out1) -> Mux/6
  Subsystem7/1(Out1) -> Mux/7
  Subsystem8/1(Out1) -> Mux/8
  Subsystem9/1(Out1) -> Mux/9
  Subsystem10/1(Out1) -> Mux/10
  Subsystem11/1(Out1) -> Mux/11
  Subsystem12/1(Out1) -> Mux/12
  Subsystem13/1(Out1) -> Mux/13
  Subsystem14/1(Out1) -> Mux/14
  Subsystem15/1(Out1) -> Mux/15
  Subsystem6/1(Out1) -> Mux/16
  Mux/1 -> MO_CV_FLT/1  "MO_CV_FLT"

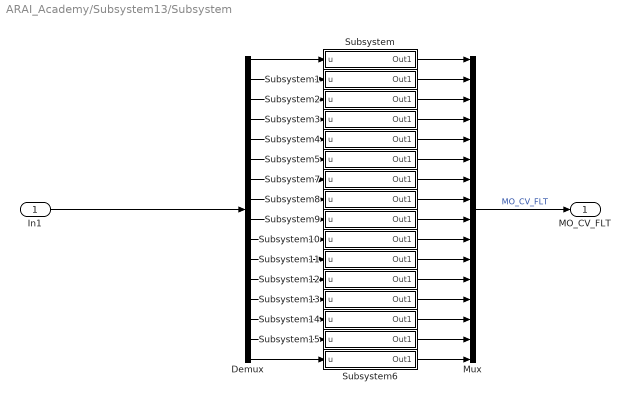
== system ARAI_Academy/Subsystem13/Subsystem ==
  In1 : Inport
  Demux : Demux  Outputs=16
  Mux : Mux  Inputs=16
  Subsystem : Subsystem
  Subsystem1 : Subsystem
  Subsystem10 : Subsystem
  Subsystem11 : Subsystem
  Subsystem12 : Subsystem
  Subsystem13 : Subsystem
  Subsystem14 : Subsystem
  Subsystem15 : Subsystem
  Subsystem2 : Subsystem
  Subsystem3 : Subsystem
  Subsystem4 : Subsystem
  Subsystem5 : Subsystem
  Subsystem6 : Subsystem
  Subsystem7 : Subsystem
  Subsystem8 : Subsystem
  Subsystem9 : Subsystem
  MO_CV_FLT : Outport
  wires:
  In1/1 -> Demux/1
  Demux/1 -> Subsystem/1(u)
  Demux/16 -> Subsystem6/1(u)
  Demux/2 -> Subsystem1/1(u)
  Demux/3 -> Subsystem2/1(u)
  Demux/4 -> Subsystem3/1(u)
  Demux/5 -> Subsystem4/1(u)
  Demux/6 -> Subsystem5/1(u)
  Demux/7 -> Subsystem7/1(u)
  Demux/8 -> Subsystem8/1(u)
  Demux/9 -> Subsystem9/1(u)
  Demux/10 -> Subsystem10/1(u)
  Demux/11 -> Subsystem11/1(u)
  Demux/12 -> Subsystem12/1(u)
  Demux/13 -> Subsystem13/1(u)
  Demux/14 -> Subsystem14/1(u)
  Demux/15 -> Subsystem15/1(u)
  Subsystem/1(Out1) -> Mux/1
  Subsystem1/1(Out1) -> Mux/2
  Subsystem2/1(Out1) -> Mux/3
  Subsystem3/1(Out1) -> Mux/4
  Subsystem4/1(Out1) -> Mux/5
  Subsystem5/1(Out1) -> Mux/6
  Subsystem7/1(Out1) -> Mux/7
  Subsystem8/1(Out1) -> Mux/8
  Subsystem9/1(Out1) -> Mux/9
  Subsystem10/1(Out1) -> Mux/10
  Subsystem11/1(Out1) -> Mux/11
  Subsystem12/1(Out1) -> Mux/12
  Subsystem13/1(Out1) -> Mux/13
  Subsystem14/1(Out1) -> Mux/14
  Subsystem15/1(Out1) -> Mux/15
  Subsystem6/1(Out1) -> Mux/16
  Mux/1 -> MO_CV_FLT/1  "MO_CV_FLT"

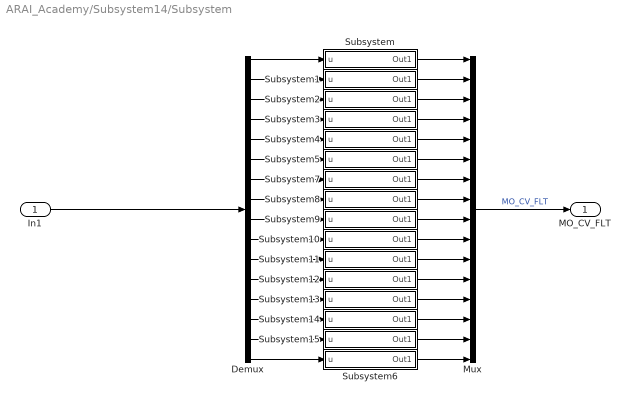
== system ARAI_Academy/Subsystem14/Subsystem ==
  In1 : Inport
  Demux : Demux  Outputs=16
  Mux : Mux  Inputs=16
  Subsystem : Subsystem
  Subsystem1 : Subsystem
  Subsystem10 : Subsystem
  Subsystem11 : Subsystem
  Subsystem12 : Subsystem
  Subsystem13 : Subsystem
  Subsystem14 : Subsystem
  Subsystem15 : Subsystem
  Subsystem2 : Subsystem
  Subsystem3 : Subsystem
  Subsystem4 : Subsystem
  Subsystem5 : Subsystem
  Subsystem6 : Subsystem
  Subsystem7 : Subsystem
  Subsystem8 : Subsystem
  Subsystem9 : Subsystem
  MO_CV_FLT : Outport
  wires:
  In1/1 -> Demux/1
  Demux/1 -> Subsystem/1(u)
  Demux/16 -> Subsystem6/1(u)
  Demux/2 -> Subsystem1/1(u)
  Demux/3 -> Subsystem2/1(u)
  Demux/4 -> Subsystem3/1(u)
  Demux/5 -> Subsystem4/1(u)
  Demux/6 -> Subsystem5/1(u)
  Demux/7 -> Subsystem7/1(u)
  Demux/8 -> Subsystem8/1(u)
  Demux/9 -> Subsystem9/1(u)
  Demux/10 -> Subsystem10/1(u)
  Demux/11 -> Subsystem11/1(u)
  Demux/12 -> Subsystem12/1(u)
  Demux/13 -> Subsystem13/1(u)
  Demux/14 -> Subsystem14/1(u)
  Demux/15 -> Subsystem15/1(u)
  Subsystem/1(Out1) -> Mux/1
  Subsystem1/1(Out1) -> Mux/2
  Subsystem2/1(Out1) -> Mux/3
  Subsystem3/1(Out1) -> Mux/4
  Subsystem4/1(Out1) -> Mux/5
  Subsystem5/1(Out1) -> Mux/6
  Subsystem7/1(Out1) -> Mux/7
  Subsystem8/1(Out1) -> Mux/8
  Subsystem9/1(Out1) -> Mux/9
  Subsystem10/1(Out1) -> Mux/10
  Subsystem11/1(Out1) -> Mux/11
  Subsystem12/1(Out1) -> Mux/12
  Subsystem13/1(Out1) -> Mux/13
  Subsystem14/1(Out1) -> Mux/14
  Subsystem15/1(Out1) -> Mux/15
  Subsystem6/1(Out1) -> Mux/16
  Mux/1 -> MO_CV_FLT/1  "MO_CV_FLT"

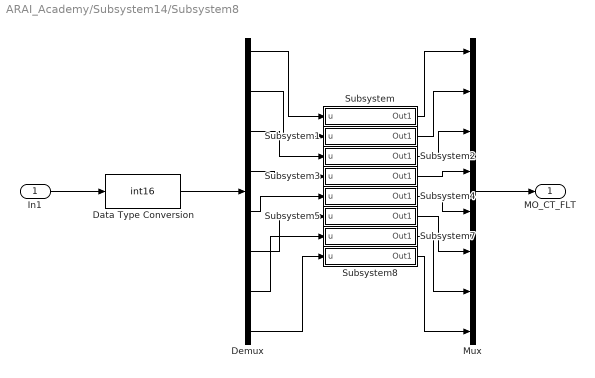
== system ARAI_Academy/Subsystem14/Subsystem8 ==
  In1 : Inport
  Data Type Conversion : DataTypeConversion  OutDataTypeStr=int16
  Demux : Demux  Outputs=8
  Mux : Mux  Inputs=8
  Subsystem : Subsystem
  Subsystem1 : Subsystem
  Subsystem2 : Subsystem
  Subsystem3 : Subsystem
  Subsystem4 : Subsystem
  Subsystem5 : Subsystem
  Subsystem7 : Subsystem
  Subsystem8 : Subsystem
  MO_CT_FLT : Outport
  wires:
  In1/1 -> Data Type Conversion/1
  Demux/1 -> Subsystem/1(u)
  Demux/2 -> Subsystem1/1(u)
  Demux/3 -> Subsystem2/1(u)
  Demux/4 -> Subsystem3/1(u)
  Demux/5 -> Subsystem4/1(u)
  Demux/6 -> Subsystem5/1(u)
  Demux/7 -> Subsystem7/1(u)
  Demux/8 -> Subsystem8/1(u)
  Subsystem/1(Out1) -> Mux/1
  Subsystem1/1(Out1) -> Mux/2
  Subsystem2/1(Out1) -> Mux/3
  Subsystem3/1(Out1) -> Mux/4
  Subsystem4/1(Out1) -> Mux/5
  Subsystem5/1(Out1) -> Mux/6
  Subsystem7/1(Out1) -> Mux/7
  Subsystem8/1(Out1) -> Mux/8
  Mux/1 -> MO_CT_FLT/1
  Data Type Conversion/1 -> Demux/1

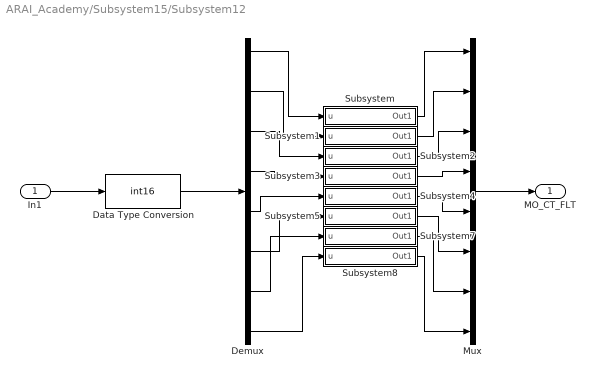
== system ARAI_Academy/Subsystem15/Subsystem12 ==
  In1 : Inport
  Data Type Conversion : DataTypeConversion  OutDataTypeStr=int16
  Demux : Demux  Outputs=8
  Mux : Mux  Inputs=8
  Subsystem : Subsystem
  Subsystem1 : Subsystem
  Subsystem2 : Subsystem
  Subsystem3 : Subsystem
  Subsystem4 : Subsystem
  Subsystem5 : Subsystem
  Subsystem7 : Subsystem
  Subsystem8 : Subsystem
  MO_CT_FLT : Outport
  wires:
  In1/1 -> Data Type Conversion/1
  Demux/1 -> Subsystem/1(u)
  Demux/2 -> Subsystem1/1(u)
  Demux/3 -> Subsystem2/1(u)
  Demux/4 -> Subsystem3/1(u)
  Demux/5 -> Subsystem4/1(u)
  Demux/6 -> Subsystem5/1(u)
  Demux/7 -> Subsystem7/1(u)
  Demux/8 -> Subsystem8/1(u)
  Subsystem/1(Out1) -> Mux/1
  Subsystem1/1(Out1) -> Mux/2
  Subsystem2/1(Out1) -> Mux/3
  Subsystem3/1(Out1) -> Mux/4
  Subsystem4/1(Out1) -> Mux/5
  Subsystem5/1(Out1) -> Mux/6
  Subsystem7/1(Out1) -> Mux/7
  Subsystem8/1(Out1) -> Mux/8
  Mux/1 -> MO_CT_FLT/1
  Data Type Conversion/1 -> Demux/1
